simulink model "PD_controller_for_TOPTD_parametric"  (R2018b)
settings: Solver=ode45  StartTime=0.0  StopTime=t_final  MaxStep=1e-3  RelTol=1e-3  EnableMultiTasking=on
values from neighbouring files (symbols this model uses):
  gain = gain_grid(i)    [main.m]    (also in main_normalized.m = final_points_normalized(1,5); mesh_generation.m = gain_mesh(i2_gain); mesh_generation_normalized.m = 1)
  Kd = x(2)    [get_step_cost_identified.m]    (also in mesh_generation.m = K(2); mesh_generation_normalized.m = 0)
  Kp = x(1)    [get_step_cost_identified.m]    (also in mesh_generation.m = K(1); mesh_generation_normalized.m = 0)
  T_body = T_body_grid(i)    [main.m]    (also in main_normalized.m = 0.2; mesh_generation.m = T_body_mesh(i2_T_body); mesh_generation_normalized.m = T_body_mesh(i2_T_body))
  T_prop = T_prop_grid(i)    [main.m]    (also in main_normalized.m = 0.015; mesh_generation.m = T_prop_mesh(i2_T_prop); mesh_generation_normalized.m = T_prop_mesh(i2_T_prop))
  tau = tau_grid(i)    [main.m]    (also in main_normalized.m = (0.1-0.001) * rand + 0.001; mesh_generation.m = tau_mesh(i2_tau); mesh_generation_normalized.m = tau_mesh(i2_tau))
libraries: simulink x1
settings Model: SimulationMode=accelerator  Creator=msa  LastModifiedBy=aaa_b
settings DataIOCC: SaveFormat=StructureWithTime
settings OptimizationCC: LifeSpan=inf
settings DebuggingCC: SolverPrmCheckMsg=warning  SFUnexpectedBacktrackingDiag=warning  SFNoUnconditionalDefaultTransitionDiag=warning  SFExecutionAtInitializationDiag=none
settings HardwareCC: ProdBitPerPointer=32  ProdBitPerSizeT=32  ProdBitPerPtrDiffT=32  ProdLargestAtomicFloat=None  ProdIntDivRoundTo=Undefined  ProdEndianess=Unspecified  ProdWordSize=32  ProdHWDeviceType=32-bit Generic
settings ModelReferenceCC: PropagateSignalLabelsOutOfModel=off
settings SFSimCC: SimUseLocalCustomCode=off
settings RTWCC: RTWUseLocalCustomCode=off
settings CodeAppCC: StateflowObjectComments=on
settings GRTTargetCC: TargetLangStandard=C89/C90 (ANSI)  GeneratePreprocessorConditionals=Disable all
settings ConfigComp: CovMetricSettings=dw  CovHtmlReporting=on  CovSaveCumulativeToWorkspaceVar=on  CovSaveSingleToWorkspaceVar=on  CovExternalEMLEnable=off  CovSFcnEnable=off

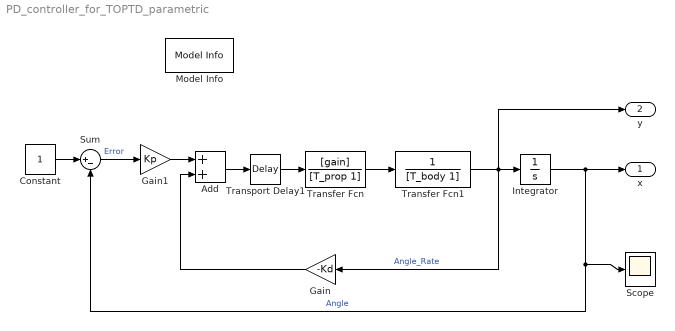
== system PD_controller_for_TOPTD_parametric ==
  Add : Sum
  Constant : Constant
  Gain : Gain  Gain=-Kd
  Gain1 : Gain  Gain=Kp
  Integrator : Integrator
  Model Info : simulink/Model-Wide Utilities/Model Info  Frame=on  DisplayStringWithTags=Model Info How should we take sensors reading WITHOUT delay  HorizontalTextAlignment=Center  LeftAlignmentValue=0.5
  Scope : Scope
  Sum : Sum  Inputs=|+-
  Transfer Fcn : TransferFcn  Numerator=[gain]  Denominator=[T_prop 1]
  Transfer Fcn1 : TransferFcn  Denominator=[T_body 1]
  Transport Delay1 : TransportDelay  DelayTime=tau
  x : Outport
  y : Outport  Port=2
  wires:
  Transfer Fcn/1 -> Transfer Fcn1/1
  Transfer Fcn1/1 -> y/1, Gain/1, Integrator/1  "Angle_Rate"
  Constant/1 -> Sum/1
  Gain/1 -> Add/2
  Gain1/1 -> Add/1
  Sum/1 -> Gain1/1  "Error"
  Integrator/1 -> Scope/1, Sum/2, x/1  "Angle"
  Add/1 -> Transport Delay1/1
  Transport Delay1/1 -> Transfer Fcn/1
